simulink model "Cancelador_de_eco"  (R2021b)
settings: Solver=VariableStepAuto  StartTime=0.0  StopTime=10.0  RelTol=1e-3
values from neighbouring files (symbols this model uses):
  T = 1    [Tempo.mat]
settings Model: Creator=duart  LastModifiedBy=duart

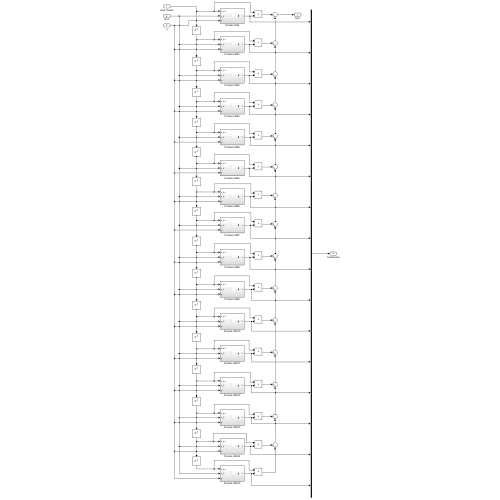
[thumbnail: Simulink's stored preview of the top-level diagram]
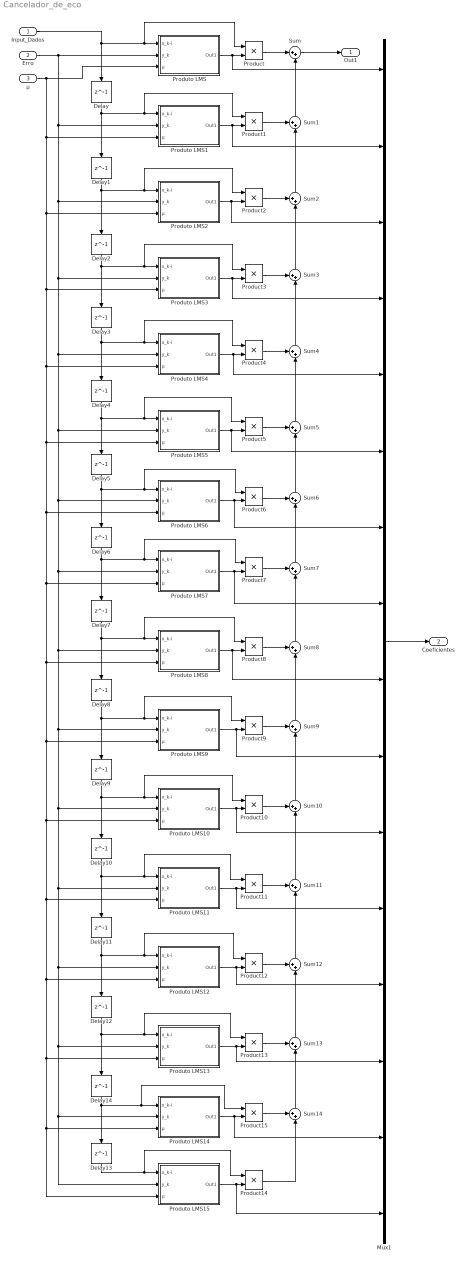
== system Cancelador_de_eco ==
  Input_Dados : Inport
  Erro : Inport  Port=2
  μ : Inport  Port=3
  Delay : Delay  DelayLength=1  InitialCondition=0  SampleTime=T
  Delay{1..14} (14 alike) : Delay  DelayLength=1  InitialCondition=0
  Mux1 : Mux  Inputs=16
  Product{,1..15} (16 alike) : Product
  Produto LMS : Subsystem
  Produto LMS1 : Subsystem
  Produto LMS10 : Subsystem
  Produto LMS11 : Subsystem
  Produto LMS12 : Subsystem
  Produto LMS13 : Subsystem
  Produto LMS14 : Subsystem
  Produto LMS15 : Subsystem
  Produto LMS2 : Subsystem
  Produto LMS3 : Subsystem
  Produto LMS4 : Subsystem
  Produto LMS5 : Subsystem
  Produto LMS6 : Subsystem
  Produto LMS7 : Subsystem
  Produto LMS8 : Subsystem
  Produto LMS9 : Subsystem
  Sum : Sum  Inputs=|++
  Sum{1..14} (14 alike) : Sum  Inputs=++|
  Out1 : Outport
  Coeficientes : Outport  Port=2
  wires:
  Input_Dados/1 -> Delay/1, Product/1, Produto LMS/1(x_k-i)
  Produto LMS/1(Out1) -> Mux1/1, Product/2
  Product/1 -> Sum/1
  Delay/1 -> Delay1/1, Product1/1, Produto LMS1/1(x_k-i)
  Produto LMS1/1(Out1) -> Mux1/2, Product1/2
  Product1/1 -> Sum1/1
  Delay1/1 -> Product2/1, Produto LMS2/1(x_k-i), Delay2/1
  Product2/1 -> Sum2/1
  Delay2/1 -> Product3/1, Produto LMS3/1(x_k-i), Delay3/1
  Product3/1 -> Sum3/1
  Delay3/1 -> Product4/1, Produto LMS4/1(x_k-i), Delay4/1
  Product4/1 -> Sum4/1
  Delay4/1 -> Product5/1, Produto LMS5/1(x_k-i), Delay5/1
  Produto LMS5/1(Out1) -> Mux1/6, Product5/2
  Product5/1 -> Sum5/1
  Delay5/1 -> Product6/1, Produto LMS6/1(x_k-i), Delay6/1
  Produto LMS6/1(Out1) -> Mux1/7, Product6/2
  Erro/1 -> Produto LMS15/2(y_k), Produto LMS14/2(y_k), Produto LMS13/2(y_k), Produto LMS12/2(y_k), Produto LMS11/2(y_k), Produto LMS10/2(y_k), Produto LMS9/2(y_k), Produto LMS8/2(y_k), Produto LMS7/2(y_k), Produto LMS6/2(y_k), Produto LMS5/2(y_k), Produto LMS4/2(y_k), Produto LMS3/2(y_k), Produto LMS2/2(y_k), Produto LMS1/2(y_k), Produto LMS/2(y_k)
  Product6/1 -> Sum6/1
  Delay6/1 -> Product7/1, Produto LMS7/1(x_k-i), Delay7/1
  Produto LMS7/1(Out1) -> Mux1/8, Product7/2
  Product7/1 -> Sum7/1
  Delay7/1 -> Delay8/1, Product8/1, Produto LMS8/1(x_k-i)
  Product8/1 -> Sum8/1
  Product9/1 -> Sum9/1
  Delay8/1 -> Delay9/1, Product9/1, Produto LMS9/1(x_k-i)
  Product10/1 -> Sum10/1
  Delay9/1 -> Delay10/1, Product10/1, Produto LMS10/1(x_k-i)
  Product11/1 -> Sum11/1
  Delay10/1 -> Delay11/1, Product11/1, Produto LMS11/1(x_k-i)
  Product12/1 -> Sum12/1
  Produto LMS12/1(Out1) -> Mux1/13, Product12/2
  Delay11/1 -> Delay12/1, Product12/1, Produto LMS12/1(x_k-i)
  Product13/1 -> Sum13/1
  Produto LMS13/1(Out1) -> Mux1/14, Product13/2
  Delay12/1 -> Delay14/1, Product13/1, Produto LMS13/1(x_k-i)
  Delay13/1 -> Product14/1, Produto LMS15/1(x_k-i)
  μ/1 -> Produto LMS14/3(μ), Produto LMS15/3(μ), Produto LMS13/3(μ), Produto LMS12/3(μ), Produto LMS11/3(μ), Produto LMS10/3(μ), Produto LMS9/3(μ), Produto LMS8/3(μ), Produto LMS7/3(μ), Produto LMS6/3(μ), Produto LMS5/3(μ), Produto LMS4/3(μ), Produto LMS3/3(μ), Produto LMS2/3(μ), Produto LMS1/3(μ), Produto LMS/3(μ)
  Sum13/1 -> Sum12/2
  Sum12/1 -> Sum11/2
  Sum11/1 -> Sum10/2
  Sum10/1 -> Sum9/2
  Sum9/1 -> Sum8/2
  Sum8/1 -> Sum7/2
  Sum7/1 -> Sum6/2
  Sum6/1 -> Sum5/2
  Sum5/1 -> Sum4/2
  Sum4/1 -> Sum3/2
  Sum3/1 -> Sum2/2
  Sum2/1 -> Sum1/2
  Sum1/1 -> Sum/2
  Sum/1 -> Out1/1
  Produto LMS2/1(Out1) -> Mux1/3, Product2/2
  Produto LMS10/1(Out1) -> Mux1/11, Product10/2
  Produto LMS15/1(Out1) -> Mux1/16, Product14/2
  Produto LMS11/1(Out1) -> Mux1/12, Product11/2
  Produto LMS9/1(Out1) -> Product9/2, Mux1/10
  Produto LMS8/1(Out1) -> Mux1/9, Product8/2
  Mux1/1 -> Coeficientes/1
  Produto LMS3/1(Out1) -> Mux1/4, Product3/2
  Produto LMS4/1(Out1) -> Mux1/5, Product4/2
  Delay14/1 -> Delay13/1, Product15/1, Produto LMS14/1(x_k-i)
  Produto LMS14/1(Out1) -> Mux1/15, Product15/2
  Sum14/1 -> Sum13/2
  Product15/1 -> Sum14/1
  Product14/1 -> Sum14/2

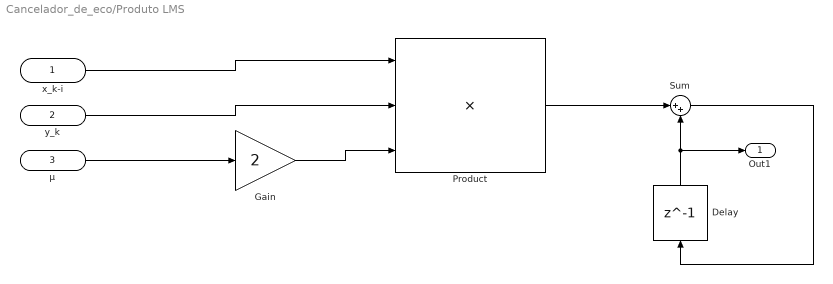
== system Cancelador_de_eco/Produto LMS ==
  x_k-i : Inport
  y_k : Inport  Port=2
  μ : Inport  Port=3
  Delay : Delay  DelayLength=1  InitialCondition=0  SampleTime=T
  Gain : Gain  Gain=2
  Product : Product  Inputs=3
  Sum : Sum  Inputs=|++
  Out1 : Outport
  wires:
  x_k-i/1 -> Product/1
  y_k/1 -> Product/2
  μ/1 -> Gain/1
  Gain/1 -> Product/3
  Product/1 -> Sum/1
  Delay/1 -> Out1/1, Sum/2
  Sum/1 -> Delay/1

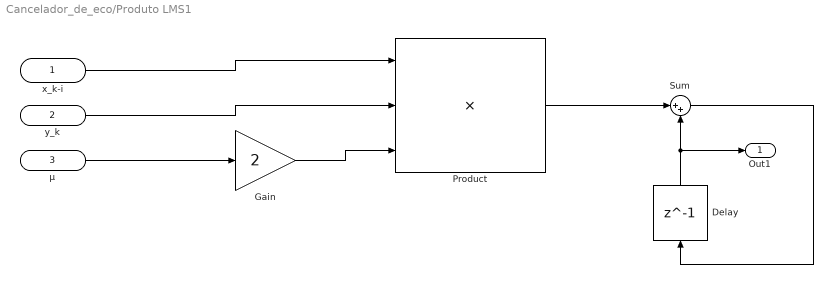
== system Cancelador_de_eco/Produto LMS1 ==
  x_k-i : Inport
  y_k : Inport  Port=2
  μ : Inport  Port=3
  Delay : Delay  DelayLength=1  InitialCondition=0  SampleTime=T
  Gain : Gain  Gain=2
  Product : Product  Inputs=3
  Sum : Sum  Inputs=|++
  Out1 : Outport
  wires:
  x_k-i/1 -> Product/1
  y_k/1 -> Product/2
  μ/1 -> Gain/1
  Gain/1 -> Product/3
  Product/1 -> Sum/1
  Delay/1 -> Out1/1, Sum/2
  Sum/1 -> Delay/1

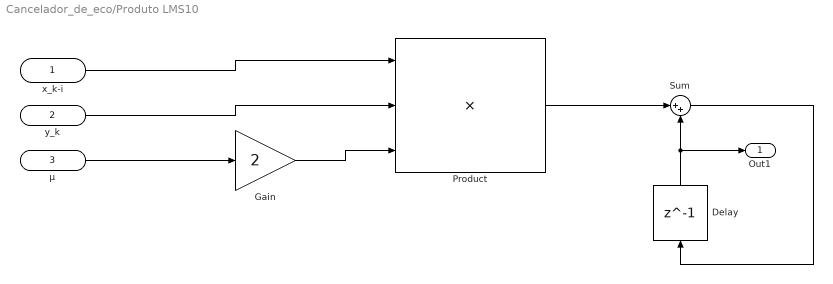
== system Cancelador_de_eco/Produto LMS10 ==
  x_k-i : Inport
  y_k : Inport  Port=2
  μ : Inport  Port=3
  Delay : Delay  DelayLength=1  InitialCondition=0  SampleTime=T
  Gain : Gain  Gain=2
  Product : Product  Inputs=3
  Sum : Sum  Inputs=|++
  Out1 : Outport
  wires:
  x_k-i/1 -> Product/1
  y_k/1 -> Product/2
  μ/1 -> Gain/1
  Gain/1 -> Product/3
  Product/1 -> Sum/1
  Delay/1 -> Out1/1, Sum/2
  Sum/1 -> Delay/1

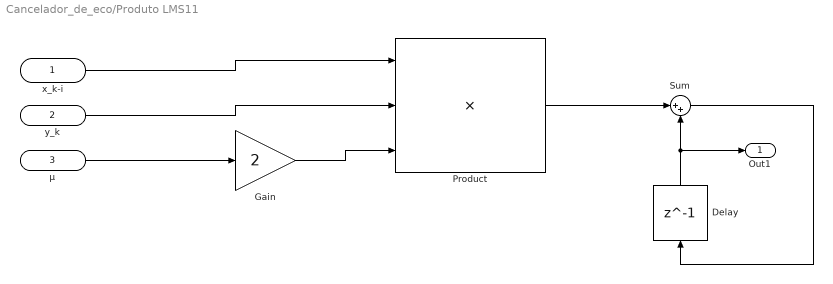
== system Cancelador_de_eco/Produto LMS11 ==
  x_k-i : Inport
  y_k : Inport  Port=2
  μ : Inport  Port=3
  Delay : Delay  DelayLength=1  InitialCondition=0  SampleTime=T
  Gain : Gain  Gain=2
  Product : Product  Inputs=3
  Sum : Sum  Inputs=|++
  Out1 : Outport
  wires:
  x_k-i/1 -> Product/1
  y_k/1 -> Product/2
  μ/1 -> Gain/1
  Gain/1 -> Product/3
  Product/1 -> Sum/1
  Delay/1 -> Out1/1, Sum/2
  Sum/1 -> Delay/1

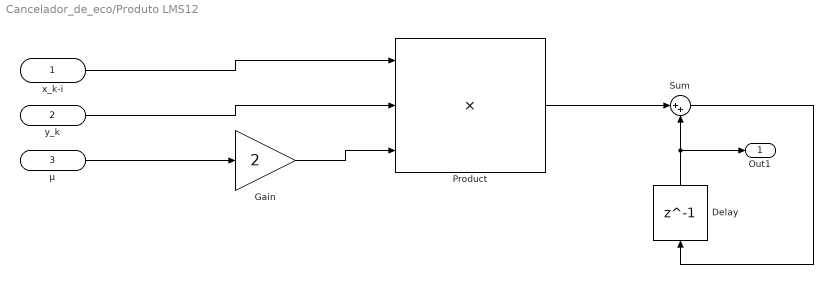
== system Cancelador_de_eco/Produto LMS12 ==
  x_k-i : Inport
  y_k : Inport  Port=2
  μ : Inport  Port=3
  Delay : Delay  DelayLength=1  InitialCondition=0  SampleTime=T
  Gain : Gain  Gain=2
  Product : Product  Inputs=3
  Sum : Sum  Inputs=|++
  Out1 : Outport
  wires:
  x_k-i/1 -> Product/1
  y_k/1 -> Product/2
  μ/1 -> Gain/1
  Gain/1 -> Product/3
  Product/1 -> Sum/1
  Delay/1 -> Out1/1, Sum/2
  Sum/1 -> Delay/1

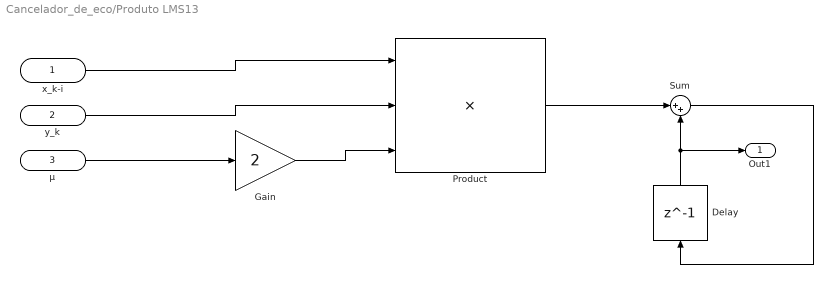
== system Cancelador_de_eco/Produto LMS13 ==
  x_k-i : Inport
  y_k : Inport  Port=2
  μ : Inport  Port=3
  Delay : Delay  DelayLength=1  InitialCondition=0  SampleTime=T
  Gain : Gain  Gain=2
  Product : Product  Inputs=3
  Sum : Sum  Inputs=|++
  Out1 : Outport
  wires:
  x_k-i/1 -> Product/1
  y_k/1 -> Product/2
  μ/1 -> Gain/1
  Gain/1 -> Product/3
  Product/1 -> Sum/1
  Delay/1 -> Out1/1, Sum/2
  Sum/1 -> Delay/1

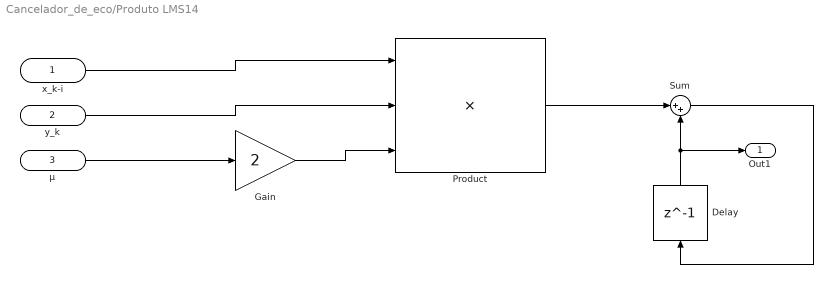
== system Cancelador_de_eco/Produto LMS14 ==
  x_k-i : Inport
  y_k : Inport  Port=2
  μ : Inport  Port=3
  Delay : Delay  DelayLength=1  InitialCondition=0  SampleTime=T
  Gain : Gain  Gain=2
  Product : Product  Inputs=3
  Sum : Sum  Inputs=|++
  Out1 : Outport
  wires:
  x_k-i/1 -> Product/1
  y_k/1 -> Product/2
  μ/1 -> Gain/1
  Gain/1 -> Product/3
  Product/1 -> Sum/1
  Delay/1 -> Out1/1, Sum/2
  Sum/1 -> Delay/1

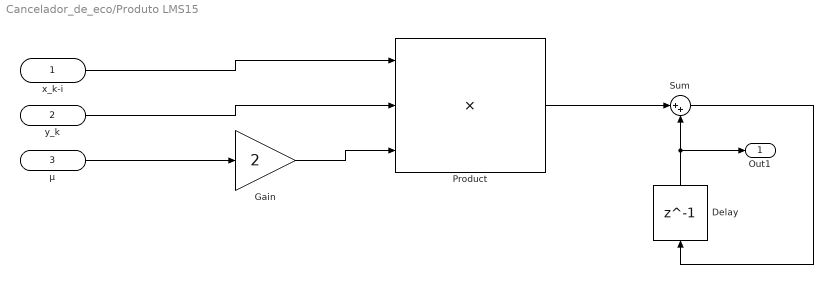
== system Cancelador_de_eco/Produto LMS15 ==
  x_k-i : Inport
  y_k : Inport  Port=2
  μ : Inport  Port=3
  Delay : Delay  DelayLength=1  InitialCondition=0  SampleTime=T
  Gain : Gain  Gain=2
  Product : Product  Inputs=3
  Sum : Sum  Inputs=|++
  Out1 : Outport
  wires:
  x_k-i/1 -> Product/1
  y_k/1 -> Product/2
  μ/1 -> Gain/1
  Gain/1 -> Product/3
  Product/1 -> Sum/1
  Delay/1 -> Out1/1, Sum/2
  Sum/1 -> Delay/1

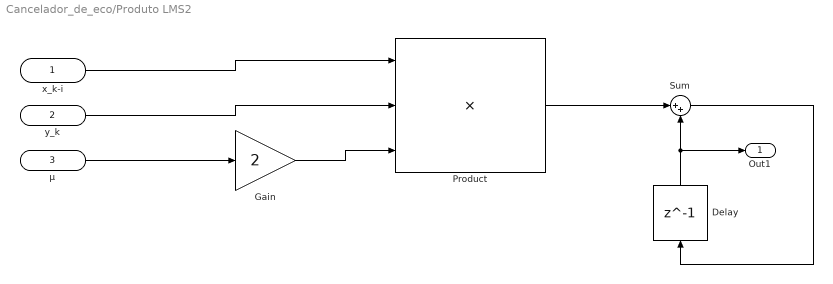
== system Cancelador_de_eco/Produto LMS2 ==
  x_k-i : Inport
  y_k : Inport  Port=2
  μ : Inport  Port=3
  Delay : Delay  DelayLength=1  InitialCondition=0  SampleTime=T
  Gain : Gain  Gain=2
  Product : Product  Inputs=3
  Sum : Sum  Inputs=|++
  Out1 : Outport
  wires:
  x_k-i/1 -> Product/1
  y_k/1 -> Product/2
  μ/1 -> Gain/1
  Gain/1 -> Product/3
  Product/1 -> Sum/1
  Delay/1 -> Out1/1, Sum/2
  Sum/1 -> Delay/1

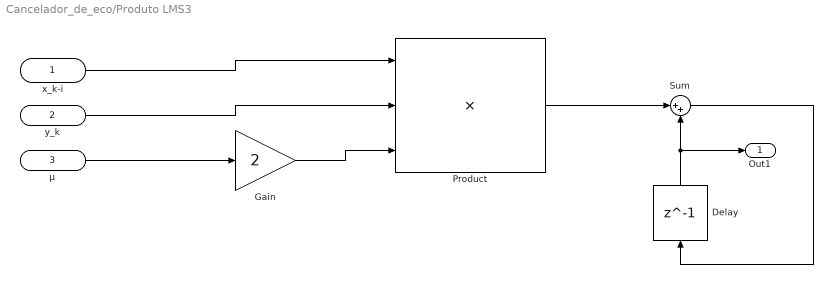
== system Cancelador_de_eco/Produto LMS3 ==
  x_k-i : Inport
  y_k : Inport  Port=2
  μ : Inport  Port=3
  Delay : Delay  DelayLength=1  InitialCondition=0  SampleTime=T
  Gain : Gain  Gain=2
  Product : Product  Inputs=3
  Sum : Sum  Inputs=|++
  Out1 : Outport
  wires:
  x_k-i/1 -> Product/1
  y_k/1 -> Product/2
  μ/1 -> Gain/1
  Gain/1 -> Product/3
  Product/1 -> Sum/1
  Delay/1 -> Out1/1, Sum/2
  Sum/1 -> Delay/1

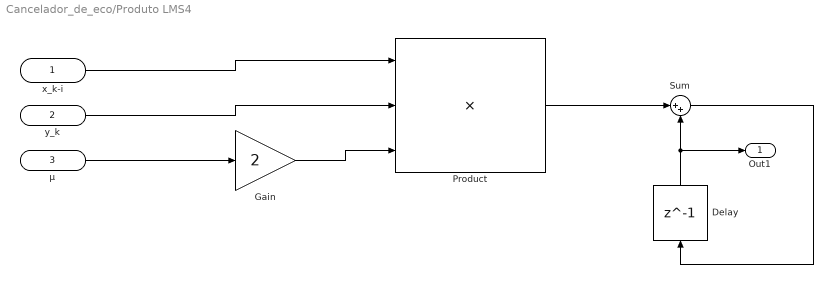
== system Cancelador_de_eco/Produto LMS4 ==
  x_k-i : Inport
  y_k : Inport  Port=2
  μ : Inport  Port=3
  Delay : Delay  DelayLength=1  InitialCondition=0  SampleTime=T
  Gain : Gain  Gain=2
  Product : Product  Inputs=3
  Sum : Sum  Inputs=|++
  Out1 : Outport
  wires:
  x_k-i/1 -> Product/1
  y_k/1 -> Product/2
  μ/1 -> Gain/1
  Gain/1 -> Product/3
  Product/1 -> Sum/1
  Delay/1 -> Out1/1, Sum/2
  Sum/1 -> Delay/1

== system Cancelador_de_eco/Produto LMS5 ==
  x_k-i : Inport
  y_k : Inport  Port=2
  μ : Inport  Port=3
  Delay : Delay  DelayLength=1  InitialCondition=0  SampleTime=T
  Gain : Gain  Gain=2
  Product : Product  Inputs=3
  Sum : Sum  Inputs=|++
  Out1 : Outport
  wires:
  x_k-i/1 -> Product/1
  y_k/1 -> Product/2
  μ/1 -> Gain/1
  Gain/1 -> Product/3
  Product/1 -> Sum/1
  Delay/1 -> Out1/1, Sum/2
  Sum/1 -> Delay/1

== system Cancelador_de_eco/Produto LMS6 ==
  x_k-i : Inport
  y_k : Inport  Port=2
  μ : Inport  Port=3
  Delay : Delay  DelayLength=1  InitialCondition=0  SampleTime=T
  Gain : Gain  Gain=2
  Product : Product  Inputs=3
  Sum : Sum  Inputs=|++
  Out1 : Outport
  wires:
  x_k-i/1 -> Product/1
  y_k/1 -> Product/2
  μ/1 -> Gain/1
  Gain/1 -> Product/3
  Product/1 -> Sum/1
  Delay/1 -> Out1/1, Sum/2
  Sum/1 -> Delay/1

== system Cancelador_de_eco/Produto LMS7 ==
  x_k-i : Inport
  y_k : Inport  Port=2
  μ : Inport  Port=3
  Delay : Delay  DelayLength=1  InitialCondition=0  SampleTime=T
  Gain : Gain  Gain=2
  Product : Product  Inputs=3
  Sum : Sum  Inputs=|++
  Out1 : Outport
  wires:
  x_k-i/1 -> Product/1
  y_k/1 -> Product/2
  μ/1 -> Gain/1
  Gain/1 -> Product/3
  Product/1 -> Sum/1
  Delay/1 -> Out1/1, Sum/2
  Sum/1 -> Delay/1

== system Cancelador_de_eco/Produto LMS8 ==
  x_k-i : Inport
  y_k : Inport  Port=2
  μ : Inport  Port=3
  Delay : Delay  DelayLength=1  InitialCondition=0  SampleTime=T
  Gain : Gain  Gain=2
  Product : Product  Inputs=3
  Sum : Sum  Inputs=|++
  Out1 : Outport
  wires:
  x_k-i/1 -> Product/1
  y_k/1 -> Product/2
  μ/1 -> Gain/1
  Gain/1 -> Product/3
  Product/1 -> Sum/1
  Delay/1 -> Out1/1, Sum/2
  Sum/1 -> Delay/1

== system Cancelador_de_eco/Produto LMS9 ==
  x_k-i : Inport
  y_k : Inport  Port=2
  μ : Inport  Port=3
  Delay : Delay  DelayLength=1  InitialCondition=0  SampleTime=T
  Gain : Gain  Gain=2
  Product : Product  Inputs=3
  Sum : Sum  Inputs=|++
  Out1 : Outport
  wires:
  x_k-i/1 -> Product/1
  y_k/1 -> Product/2
  μ/1 -> Gain/1
  Gain/1 -> Product/3
  Product/1 -> Sum/1
  Delay/1 -> Out1/1, Sum/2
  Sum/1 -> Delay/1
